simulink model "Example"  (R2021b)
settings: Solver=ode1  StartTime=0.0  StopTime=40  FixedStep=0.001  RelTol=1e-3
PreLoadFcn:
  | run('Example_init.m')
values from neighbouring files (symbols this model uses):
  A = BWB.lat.A    [SMC_Example_init.m]
  B = BWB.lat.B    [SMC_Example_init.m]
  C = eye(n)    [SMC_Example_init.m]
  Cc = [1 0 0 0 ... (first row only)    [SMC_Example_init.m]
  D = zeros(p,m)    [SMC_Example_init.m]
  x0 = zeros(1,n)    [SMC_Example_init.m]
libraries: SMC x1
settings Model: Creator=lev201  LastModifiedBy=w.schwamm
settings SolverCC: AlgebraicLoopSolver=TrustRegion
settings DataIOCC: ReturnWorkspaceOutputs=off
settings DebuggingCC: SFMachineParentedDataDiag=warning  ArithmeticOperatorsInVariantConditions=warning
settings SFSimCC: SimUseLocalCustomCode=off  CustomCodeUndefinedFunction=UseInterfaceOnly
settings RTWCC: RTWUseLocalCustomCode=off

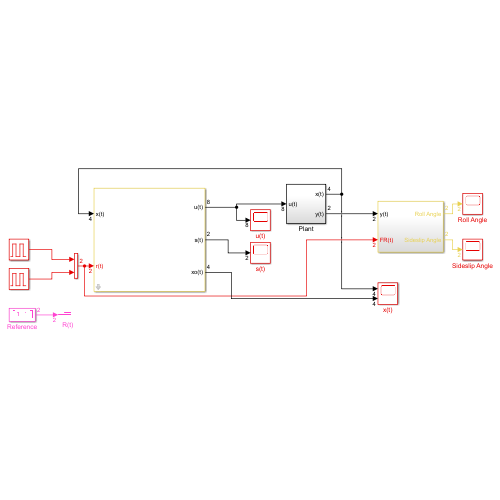
[thumbnail: Simulink's stored preview of the top-level diagram]
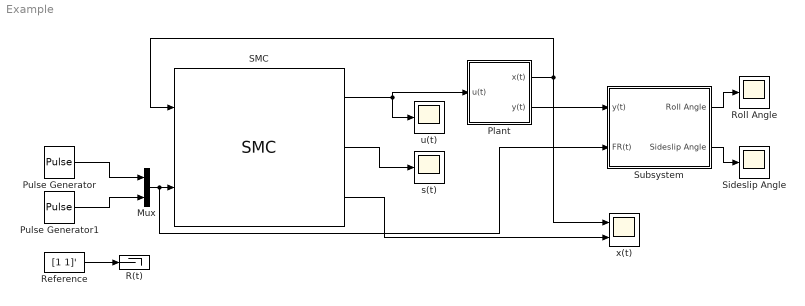
== system Example ==
  Mux : Mux  Inputs=2
  Plant : Subsystem
  Pulse Generator : DiscretePulseGenerator  PulseType=Time based  Period=20  PulseWidth=50
  Pulse Generator1 : DiscretePulseGenerator  PulseType=Time based  Period=20  PulseWidth=50  PhaseDelay=10
  R(t) : Terminator
  Reference : Constant  Value=[1 1]'
  Roll Angle : Scope
  SMC : SMC/SMC  ia=on  obs=on  adpt=off  shs=on  shxo=on  shadpt=off  A=A  B=B  Cc=Cc  x0=x0  obstype=Walcott_Zak  z0=zeros(1,length(x0))  Q=Q  rho=5  delta=0.01  eps=0  C0=1  PC=1  K0=1  PK=1  Qi=Qi  Fil=off  Filter=F  FRt=on  rhoo=15  deltao=0.01  epso=0
  Sideslip Angle : Scope
  Subsystem : Subsystem
  s(t) : Scope
  u(t) : Scope
  x(t) : Scope  NumInputPorts=2
  wires:
  Plant/2(y(t)) -> Subsystem/1(y(t))
  SMC/1 -> Plant/1(u(t)), u(t)/1
  Subsystem/1(Roll Angle) -> Roll Angle/1
  Subsystem/2(Sideslip Angle) -> Sideslip Angle/1
  Pulse Generator/1 -> Mux/1
  Pulse Generator1/1 -> Mux/2
  SMC/2 -> s(t)/1
  Plant/1(x(t)) -> x(t)/1, SMC/1
  Reference/1 -> R(t)/1
  Mux/1 -> Subsystem/2(FR(t)), SMC/2
  SMC/3 -> x(t)/2

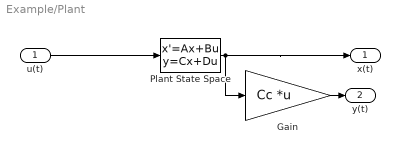
== system Example/Plant ==
  u(t) : Inport
  Gain : Gain  Gain=Cc  Multiplication=Matrix(K*u) (u vector)
  Plant State Space : StateSpace  A=A  B=B  C=C  D=D  InitialCondition=[0 0.1 0 0]
  x(t) : Outport  VectorParamsAs1DForOutWhenUnconnected=off
  y(t) : Outport  Port=2  VectorParamsAs1DForOutWhenUnconnected=off
  wires:
  u(t)/1 -> Plant State Space/1
  Plant State Space/1 -> Gain/1, x(t)/1
  Gain/1 -> y(t)/1

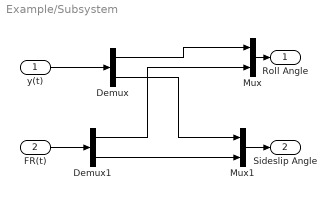
== system Example/Subsystem ==
  y(t) : Inport
  FR(t) : Inport  Port=2
  Demux : Demux  Outputs=2
  Demux1 : Demux  Outputs=2
  Mux : Mux  Inputs=2
  Mux1 : Mux  Inputs=2
  Roll Angle : Outport  VectorParamsAs1DForOutWhenUnconnected=off
  Sideslip Angle : Outport  Port=2  VectorParamsAs1DForOutWhenUnconnected=off
  wires:
  y(t)/1 -> Demux/1
  Demux/1 -> Mux/1
  Mux/1 -> Roll Angle/1
  Mux1/1 -> Sideslip Angle/1
  Demux/2 -> Mux1/1
  FR(t)/1 -> Demux1/1
  Demux1/1 -> Mux/2
  Demux1/2 -> Mux1/2
